simulink model "Shin_com"  (R2024a)
settings: Solver=VariableStepAuto  StartTime=0.0  StopTime=10.0  RelTol=1e-3
undefined symbols (not defined in the file): route1_waypoint_x, route1_waypoint_y, route2_waypoint_x, route2_waypoint_y, route3_waypoint_x, route3_waypoint_y, route4_waypoint_x, route4_waypoint_y, route5_waypoint_x, route5_waypoint_y
libraries: CarMaker4SL x162, slpidlib x4, robotalgslib x1, matrix_library x1
(part 1 of 4)
settings Model: Creator=User  LastModifiedBy=User

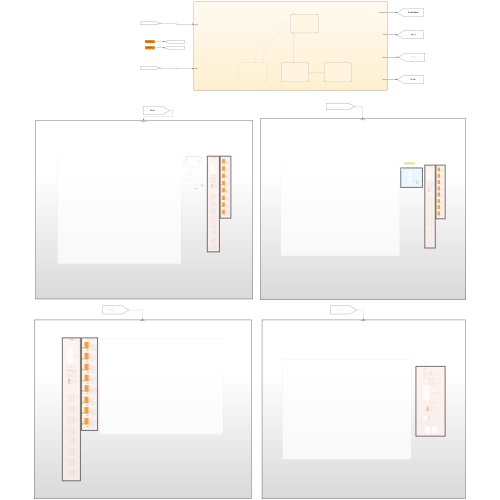
[thumbnail: Simulink's stored preview of the top-level diagram]
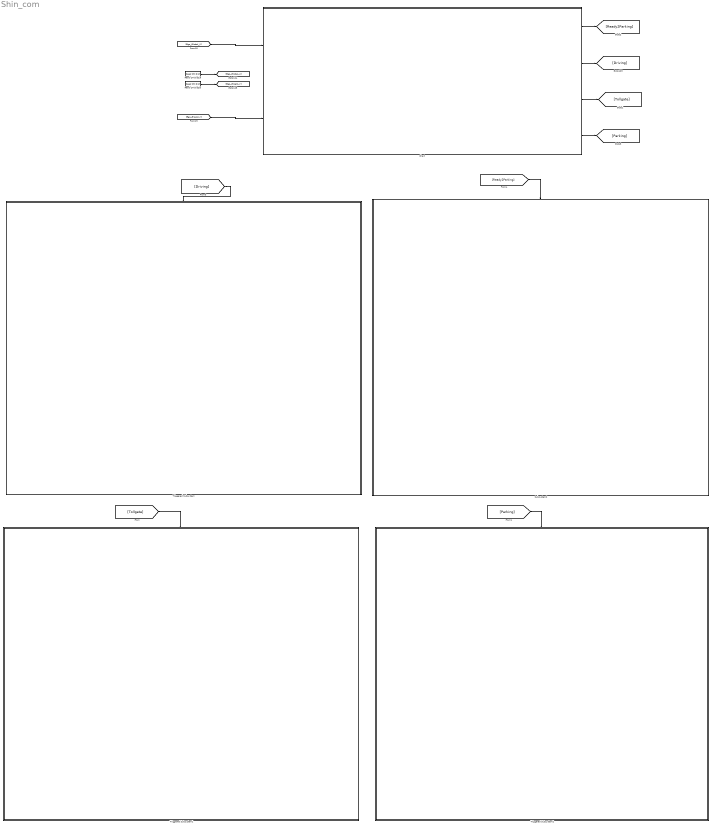
== system Shin_com ==
  Chart : Stateflow chart  TreatAsAtomicUnit=on
  Read CM Dict19 : CarMaker4SL/Read CM Dict  xname=Car.Fr1.tx  xsync=off  xstime=Inherited
  Read CM Dict20 : CarMaker4SL/Read CM Dict  xname=Car.Fr1.ty  xsync=off  xstime=Inherited
  Subsystem2 : Subsystem
  Triggered Subsystem : Subsystem  TreatAsAtomicUnit=on
  Triggered Subsystem1 : Subsystem  TreatAsAtomicUnit=on
  Triggered Subsystem2 : Subsystem  TreatAsAtomicUnit=on
  wires:
  Chart/3(tollgate()) -> [Tollgate]
  Read CM Dict20/1 -> [Ego_Gloabl_Y]
  [Driving] -> Triggered Subsystem/Trigger
  Chart/1(ready2parking()) -> [Ready2Parking]
  Chart/2(driving()) -> [Driving]
  [Ready2Parking] -> Subsystem2/Trigger
  [Ego_Global_X] -> Chart/1(global_X)
  [Ego_Gloabl_Y] -> Chart/2(global_Y)
  [Parking] -> Triggered Subsystem2/Trigger
  Chart/4(parking()) -> [Parking]
  Read CM Dict19/1 -> [Ego_Global_X]
  [Tollgate] -> Triggered Subsystem1/Trigger

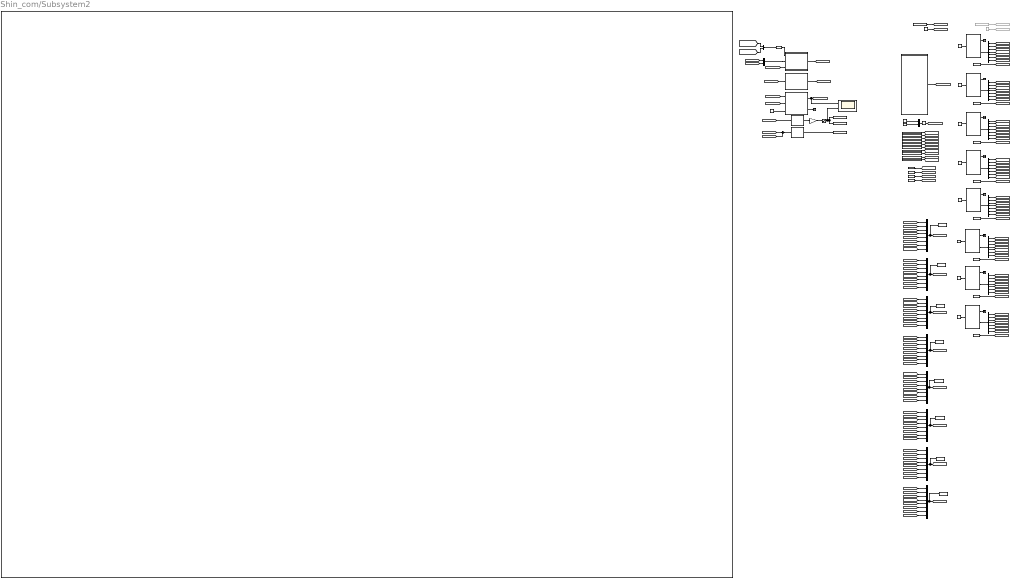
== system Shin_com/Subsystem2 ==
  note: Rpute 5
  note: *** Final Project ***
      |
      | Scenario:
      | Input:
      | Output:
      | 제어기 10ms / 다익스트라 1s
  note: Traffic Size
      | Length: 4.47
      | Width: 1.97
      | Height: 1.12
  note: Traffic Size
      | Length: 4.47
      | Width: 1.97
      | Height: 1.12
  note: Traffic Size
      | Length: 4.47
      | Width: 1.97
      | Height: 1.12
  note: Traffic Size
      | Length: 4.47
      | Width: 1.97
      | Height: 1.12
  note: Do Not Modify !!
  note: Traffic Size
      | Length: 4.47
      | Width: 1.97
      | Height: 1.12
  note: Traffic Size
      | Length: 4.47
      | Width: 1.97
      | Height: 1.12
  note: Do Not Modify !!
  note: Traffic Size
      | Length: 4.47
      | Width: 1.97
      | Height: 1.12
  note: Traffic Size
      | Length: 4.47
      | Width: 1.97
      | Height: 1.12
  Trigger : TriggerPort  TriggerType=function-call  VariantControl=(inherit)  PortDimensions=1
      mask Display: image('20210726111455075uqcv.jpg');
  Bus Selector{3..10} (8 alike) : BusSelector  OutputSignals=t_0 x,t_0 y,v_0 x,v_0 y,a_0 x,a_0 y,r_zyx z
  Constant : Constant  Value=0.5
  Constant11 : Constant  Value=28
  Constant12 : Constant  Value=route1_waypoint_y.Data
  Constant13 : Constant  Value=route2_waypoint_y.Data
  Constant14 : Constant  Value=route2_waypoint_x.Data
  Constant15 : Constant  Value=route1_waypoint_x.Data
  Constant16 : Constant  Value=route3_waypoint_y.Data
  Constant17 : Constant  Value=route3_waypoint_x.Data
  Constant18 : Constant  Value=route4_waypoint_y.Data
  Constant19 : Constant  Value=route4_waypoint_x.Data
  Constant20 : Constant  Value=route5_waypoint_y.Data
  Constant21 : Constant  Value=route5_waypoint_x.Data
  Constant22 : Constant  Value=23
  Constant23 : Constant  Value=20/3.6
  Constant25 : Constant  Value=11.5
  Constant26 : Constant  Value=24
  Constant27 : Constant  Value=25
  Constant28 : Constant  Value=26
  Constant29 : Constant  Value=27
  Constant6 : Constant  Commented=on  Value=20/3.6
  Constant7 : Constant  Value=21
  Constant8 : Constant  Value=2.48
  Constant9 : Constant  Value=22
  Gain : Gain  Gain=pi/180
  Goto31 : Goto  Commented=on  GotoTag=CrossTrackError
  Goto64 : Goto  Commented=on  GotoTag=Target_Speed
  MATLAB Function4 : MATLAB Function  TreatAsAtomicUnit=on
  "MATLAB Function4 " : MATLAB Function  TreatAsAtomicUnit=on
  MATLAB Function7 : MATLAB Function  TreatAsAtomicUnit=on
  Mux{,1..2,5..9} (8 alike) : Mux  Inputs=8
  Mux12 : Mux  Inputs=2
  Mux13 : Mux  Inputs=2
  Mux4 : Mux  Inputs=2
  PID Controller2 : slpidlib/PID Controller  Controller=PID  Form=Parallel  TimeDomain=Discrete-time  UseExternalTs=off  SampleTime=-1  IntegratorMethod=Forward Euler  FilterMethod=Forward Euler  ControllerParametersSource=internal  P=1  I=0.0  UseKiTs=off  D=0  UseExternalDerivativeSource=off  N=100  UseFilter=on  TunerSelectOption=Transfer Function Based (PID Tuner App)  InitialConditionSource=internal  InitialConditionForIntegrator=0  InitialConditionForFilter=0  DifferentiatorICPrevScaledInput=0  ExternalReset=none  TrackingMode=off  Kt=1  LimitOutput=off  SatLimitsSource=internal  UpperSaturationLimit=inf  LowerSaturationLimit=-inf  LinearizeAsGain=on  AntiWindupMode=none  Kb=1  LimitIntegrator=off  UpperIntegratorSaturationLimit=inf  LowerIntegratorSaturationLimit=-inf  POutMin=[]  POutMax=[]  IOutMin=[]  IOutMax=[]  DOutMin=[]  DOutMax=[]  NOutMin=[]  NOutMax=[]  SumOutMin=[]  SumOutMax=[]  SaturationOutMin=[]  SaturationOutMax=[]  PParamMin=[]  PParamMax=[]  IParamMin=[]  IParamMax=[]  DParamMin=[]  DParamMax=[]  NParamMin=[]  NParamMax=[]  KbParamMin=[]  KbParamMax=[]  KtParamMin=[]  KtParamMax=[]  KbOutMin=[]  KbOutMax=[]  KtOutMin=[]  KtOutMax=[]  IntegratorOutMin=[]  IntegratorOutMax=[]  FilterOutMin=[]  FilterOutMax=[]  SumI1OutMin=[]  SumI1OutMax=[]  SumI2OutMin=[]  SumI2OutMax=[]  SumI3OutMin=[]  SumI3OutMax=[]  SumI4OutMin=[]  SumI4OutMax=[]  SumDOutMin=[]  SumDOutMax=[]  DifferentiatorOutMin=[]  DifferentiatorOutMax=[]  FilterDiffOutCoefMin=[]  FilterDiffOutCoefMax=[]  ReciprocalOutMin=[]  ReciprocalOutMax=[]  SumDenOutMin=[]  SumDenOutMax=[]  SumNumOutMin=[]  SumNumOutMax=[]  DivideOutMin=[]  DivideOutMax=[]  UdiffTsProdOutMin=[]  UdiffTsProdOutMax=[]  NTsProdOutMin=[]  NTsProdOutMax=[]  UintegralTsProdOutMin=[]  UintegralTsProdOutMax=[]  UngainTsProdOutMin=[]  UngainTsProdOutMax=[]  ClampingZeroOutDataTypeStr=Inherit: Inherit via back propagation  ClampingZeroOutMin=[]  ClampingZeroOutMax=[]  FilterDenConstantOutDataTypeStr=Inherit: Inherit via back propagation  FilterDenConstantOutMin=[]  FilterDenConstantOutMax=[]  PCopyOutDataTypeStr=Inherit: Inherit via back propagation  PCopyOutMin=[]  PCopyOutMax=[]  NCopyOutDataTypeStr=Inherit: Inherit via back propagation  NCopyOutMin=[]  NCopyOutMax=[]  IntegratorContinuousStateAttributes=''  IntegratorStateMustResolveToSignalObject=off  IntegratorRTWStateStorageClass=Auto  FilterContinuousStateAttributes=''  FilterStateMustResolveToSignalObject=off  FilterRTWStateStorageClass=Auto  ParallelPVariant=InternalParameters  IdealPVariant=Disabled  IVariant=InternalParameters  DVariant=InternalParameters  IntegratorVariant=Discrete  SatVariant=Disabled  AWVariant=Passthrough  PCopyVariant=Disabled  TRVariant=Disabled  FdbkBlocksVariant=Forward  IdealPFdbkVariant=Disabled  SatFdbkVariant=Disabled  DerivativeFilterVariant=ForwardEulerFilter  NVariant=InternalParameters  NCopyVariant=Disabled  FilterICVariant=InternalICsFilter  IntegratorICVariant=InternalICs  ExternalResetVariant=Disabled  TRSumVariant=Passthrough  SumFdbkVariant=Disabled  SumVariant=Sum_PID  TsampFilterVariant=InternalTs  TsampNgainVariant=Passthrough  TsampIntegralVariant=Disabled_SignalSpec  ExternalSaturationOutDataTypeStr=Inherit: Same as second input  DerivativeSourceVariant=ErrorSignal
  PID Controller3 : slpidlib/PID Controller  Controller=PID  Form=Parallel  TimeDomain=Discrete-time  UseExternalTs=off  SampleTime=-1  IntegratorMethod=Forward Euler  FilterMethod=Forward Euler  ControllerParametersSource=internal  P=10  I=0  UseKiTs=off  D=0.1  UseExternalDerivativeSource=off  N=20  UseFilter=on  TunerSelectOption=Transfer Function Based (PID Tuner App)  InitialConditionSource=internal  InitialConditionForIntegrator=0  InitialConditionForFilter=0  DifferentiatorICPrevScaledInput=0  ExternalReset=none  TrackingMode=off  Kt=1  LimitOutput=off  SatLimitsSource=internal  UpperSaturationLimit=inf  LowerSaturationLimit=-inf  LinearizeAsGain=on  AntiWindupMode=none  Kb=1  LimitIntegrator=off  UpperIntegratorSaturationLimit=inf  LowerIntegratorSaturationLimit=-inf  POutMin=[]  POutMax=[]  IOutMin=[]  IOutMax=[]  DOutMin=[]  DOutMax=[]  NOutMin=[]  NOutMax=[]  SumOutMin=[]  SumOutMax=[]  SaturationOutMin=[]  SaturationOutMax=[]  PParamMin=[]  PParamMax=[]  IParamMin=[]  IParamMax=[]  DParamMin=[]  DParamMax=[]  NParamMin=[]  NParamMax=[]  KbParamMin=[]  KbParamMax=[]  KtParamMin=[]  KtParamMax=[]  KbOutMin=[]  KbOutMax=[]  KtOutMin=[]  KtOutMax=[]  IntegratorOutMin=[]  IntegratorOutMax=[]  FilterOutMin=[]  FilterOutMax=[]  SumI1OutMin=[]  SumI1OutMax=[]  SumI2OutMin=[]  SumI2OutMax=[]  SumI3OutMin=[]  SumI3OutMax=[]  SumI4OutMin=[]  SumI4OutMax=[]  SumDOutMin=[]  SumDOutMax=[]  DifferentiatorOutMin=[]  DifferentiatorOutMax=[]  FilterDiffOutCoefMin=[]  FilterDiffOutCoefMax=[]  ReciprocalOutMin=[]  ReciprocalOutMax=[]  SumDenOutMin=[]  SumDenOutMax=[]  SumNumOutMin=[]  SumNumOutMax=[]  DivideOutMin=[]  DivideOutMax=[]  UdiffTsProdOutMin=[]  UdiffTsProdOutMax=[]  NTsProdOutMin=[]  NTsProdOutMax=[]  UintegralTsProdOutMin=[]  UintegralTsProdOutMax=[]  UngainTsProdOutMin=[]  UngainTsProdOutMax=[]  ClampingZeroOutDataTypeStr=Inherit: Inherit via back propagation  ClampingZeroOutMin=[]  ClampingZeroOutMax=[]  FilterDenConstantOutDataTypeStr=Inherit: Inherit via back propagation  FilterDenConstantOutMin=[]  FilterDenConstantOutMax=[]  PCopyOutDataTypeStr=Inherit: Inherit via back propagation  PCopyOutMin=[]  PCopyOutMax=[]  NCopyOutDataTypeStr=Inherit: Inherit via back propagation  NCopyOutMin=[]  NCopyOutMax=[]  IntegratorContinuousStateAttributes=''  IntegratorStateMustResolveToSignalObject=off  IntegratorRTWStateStorageClass=Auto  FilterContinuousStateAttributes=''  FilterStateMustResolveToSignalObject=off  FilterRTWStateStorageClass=Auto  ParallelPVariant=InternalParameters  IdealPVariant=Disabled  IVariant=InternalParameters  DVariant=InternalParameters  IntegratorVariant=Discrete  SatVariant=Disabled  AWVariant=Passthrough  PCopyVariant=Disabled  TRVariant=Disabled  FdbkBlocksVariant=Forward  IdealPFdbkVariant=Disabled  SatFdbkVariant=Disabled  DerivativeFilterVariant=ForwardEulerFilter  NVariant=InternalParameters  NCopyVariant=Disabled  FilterICVariant=InternalICsFilter  IntegratorICVariant=InternalICs  ExternalResetVariant=Disabled  TRSumVariant=Passthrough  SumFdbkVariant=Disabled  SumVariant=Sum_PID  TsampFilterVariant=InternalTs  TsampNgainVariant=Passthrough  TsampIntegralVariant=Disabled_SignalSpec  ExternalSaturationOutDataTypeStr=Inherit: Same as second input  DerivativeSourceVariant=ErrorSignal
  Read CM Dict10 : CarMaker4SL/Read CM Dict  xname=Car.Fr1.tx  xsync=off  xstime=Inherited
  Read CM Dict11 : CarMaker4SL/Read CM Dict  xname=Car.Fr1.ty  xsync=off  xstime=Inherited
  Read CM Dict12 : CarMaker4SL/Read CM Dict  xname=Car.Fr1.rz  xsync=off  xstime=Inherited
  Read CM Dict13 : CarMaker4SL/Read CM Dict  xname=Car.v  xsync=off  xstime=Inherited
  Read CM Dict14 : CarMaker4SL/Read CM Dict  xname=Traffic.T24.rzv  xsync=off  xstime=Inherited
  Read CM Dict15 : CarMaker4SL/Read CM Dict  xname=Traffic.T25.rzv  xsync=off  xstime=Inherited
  Read CM Dict16 : CarMaker4SL/Read CM Dict  xname=Traffic.T26.rzv  xsync=off  xstime=Inherited
  Read CM Dict17 : CarMaker4SL/Read CM Dict  xname=Traffic.T27.rzv  xsync=off  xstime=Inherited
  Read CM Dict18 : CarMaker4SL/Read CM Dict  xname=Traffic.T28.rzv  xsync=off  xstime=Inherited
  Read CM Dict5 : CarMaker4SL/Read CM Dict  Commented=on  xname=Car.Road.Path.DevDist  xsync=off  xstime=Inherited
  Read CM Dict6 : CarMaker4SL/Read CM Dict  xname=Traffic.T21.rzv  xsync=off  xstime=Inherited
  Read CM Dict7 : CarMaker4SL/Read CM Dict  xname=Traffic.T22.rzv  xsync=off  xstime=Inherited
  Read CM Dict8 : CarMaker4SL/Read CM Dict  xname=Traffic.T23.rzv  xsync=off  xstime=Inherited
  Read CM Dict9 : CarMaker4SL/Read CM Dict  xname=Car.Road.Path.DevDist  xsync=off  xstime=Inherited
  Reshape2 : Reshape  OutputDimensionality=Row vector (2-D)  OutputDimensions=[2,2]
  Reshape3 : Reshape  OutputDimensionality=Customize  OutputDimensions=[201, 2]
  Saturation1 : Saturate  UpperLimit=2  LowerLimit=-2
  Scope : Scope  NumInputPorts=2
  Subsystem1 : Subsystem
  Sum : Sum  Inputs=|+-
  Terminator{,3..9,11} (9 alike) : Terminator
  To Workspace : ToWorkspace  VariableName=obs_x2  SaveFormat=Timeseries  SampleTime=-1
  To Workspace1 : ToWorkspace  VariableName=obs_Vx2  SaveFormat=Timeseries  SampleTime=-1
  To Workspace2 : ToWorkspace  VariableName=obs_YawRate2  SaveFormat=Timeseries  SampleTime=-1
  To Workspace3 : ToWorkspace  VariableName=obs_Ax2  SaveFormat=Timeseries  SampleTime=-1
  To Workspace4 : ToWorkspace  VariableName=obs_y2  SaveFormat=Timeseries  SampleTime=-1
  To Workspace5 : ToWorkspace  VariableName=obs_Vy2  SaveFormat=Timeseries  SampleTime=-1
  To Workspace6 : ToWorkspace  VariableName=obs_Yaw2  SaveFormat=Timeseries  SampleTime=-1
  To Workspace7 : ToWorkspace  VariableName=obs_Ay2  SaveFormat=Timeseries  SampleTime=-1
  Traffic Object10 : CarMaker4SL/Traffic Object  xname=T28  ximode=Traffic Id  xstime=Inherited
      settings: SourceProductName=CarMaker4SL
  Traffic Object3 : CarMaker4SL/Traffic Object  xname=T21  ximode=Traffic Id  xstime=Inherited
      settings: SourceProductName=CarMaker4SL
  Traffic Object4 : CarMaker4SL/Traffic Object  xname=T22  ximode=Traffic Id  xstime=Inherited
      settings: SourceProductName=CarMaker4SL
  Traffic Object5 : CarMaker4SL/Traffic Object  xname=T23  ximode=Traffic Id  xstime=Inherited
      settings: SourceProductName=CarMaker4SL
  Traffic Object6 : CarMaker4SL/Traffic Object  xname=T24  ximode=Traffic Id  xstime=Inherited
      settings: SourceProductName=CarMaker4SL
  Traffic Object7 : CarMaker4SL/Traffic Object  xname=T25  ximode=Traffic Id  xstime=Inherited
      settings: SourceProductName=CarMaker4SL
  Traffic Object8 : CarMaker4SL/Traffic Object  xname=T26  ximode=Traffic Id  xstime=Inherited
      settings: SourceProductName=CarMaker4SL
  Traffic Object9 : CarMaker4SL/Traffic Object  xname=T27  ximode=Traffic Id  xstime=Inherited
      settings: SourceProductName=CarMaker4SL
  Write CM Dict1 : CarMaker4SL/Write CM Dict  xname=AccelCtrl.DesiredAx  xsync=off
  Write CM Dict2 : CarMaker4SL/Write CM Dict  xname=Car.CFL.rz_ext  xsync=off
  Write CM Dict3 : CarMaker4SL/Write CM Dict  xname=Car.CFR.rz_ext  xsync=off
  wires:
  [Ego_Gloabl_Y] -> Mux13/2
  Mux12/1 -> Reshape3/1
  Reshape3/1 -> "MATLAB Function4 "/1(waypoints)
  [Ego_Global_X] -> Mux13/1
  [route5_waypoint_x] -> Mux12/1
  "MATLAB Function4 "/1(local_waypoints_) -> [Local_Points]
  [route5_waypoint_y] -> Mux12/2
  Mux13/1 -> "MATLAB Function4 "/2(vehicle_position)
  [Ego_Yaw] -> "MATLAB Function4 "/3(head)
  MATLAB Function7/1(poly_coeff) -> [Coefficients]
  [Local_Points] -> MATLAB Function7/1(local_waypoints)
  [Coefficients] -> MATLAB Function4/1(poly_coeff)
  MATLAB Function4/1(lateral_error) -> Scope/1, [LateralError]  "LatelralError"
  [LateralError] -> PID Controller3/1
  [Traffic27_Ax] -> Mux8/7
  Bus Selector10/1 -> [Traffic28_Global_X]  "<t_0 x>"
  Constant25/1 -> Mux4/2
  [Traffic23_Ay] -> Mux9/3
  [Traffic25_Yaw] -> Mux7/5
  Constant7/1 -> Traffic Object3/1
  Read CM Dict15/1 -> [Traffic25_YawRate]
  [Traffic23_Ax] -> Mux8/3
  Bus Selector6/3 -> [Traffic24_Vx]  "<v_0 x>"
  [Traffic23_Vy] -> Mux5/3
  Bus Selector7/5 -> [Traffic25_Ax]  "<a_0 x>"
  Bus Selector10/3 -> [Traffic28_Vx]  "<v_0 x>"
  Bus Selector3/6 -> [Traffic21_Ay]  "<a_0 y>"
  Constant20/1 -> [route5_waypoint_y]
  Constant27/1 -> Traffic Object7/1
  [Traffic26_Yaw] -> Mux7/6
  Subsystem1/1(Traffic_Info) -> [Traffic_Info]
  Bus Selector8/2 -> [Traffic26_Global_Y]  "<t_0 y>"
  Constant9/1 -> Traffic Object4/1
  Mux8/1 -> To Workspace3/1, [obs_Ax]
  Constant21/1 -> [route5_waypoint_x]
  Bus Selector5/4 -> [Traffic23_Vy]  "<v_0 y>"
  Read CM Dict7/1 -> [Traffic22_YawRate]
  Bus Selector7/3 -> [Traffic25_Vx]  "<v_0 x>"
  [Traffic25_Vx] -> Mux2/5
  Constant16/1 -> [route3_waypoint_y]
  Constant18/1 -> [route4_waypoint_y]
  [Traffic27_Vy] -> Mux5/7
  Traffic Object8/1 -> Terminator8/1
  [Traffic23_Global_X] -> Mux/3
  Constant19/1 -> [route4_waypoint_x]
  [Traffic21_Global_X] -> Mux/1
  Traffic Object4/2 -> Bus Selector4/1
  [Traffic25_YawRate] -> Mux6/5
  Bus Selector9/5 -> [Traffic27_Ax]  "<a_0 x>"
  Bus Selector8/5 -> [Traffic26_Ax]  "<a_0 x>"
  Read CM Dict11/1 -> [Ego_Gloabl_Y]
  [Traffic28_Global_X] -> Mux/8
  Read CM Dict16/1 -> [Traffic26_YawRate]
  Traffic Object6/1 -> Terminator6/1
  [Traffic28_Global_Y] -> Mux1/8
  Mux2/1 -> To Workspace1/1, [obs_Vx]
  [Traffic24_Vx] -> Mux2/4
  Constant17/1 -> [route3_waypoint_x]
  [Traffic25_Vy] -> Mux5/5
  [Traffic21_Vx] -> Mux2/1
  Read CM Dict6/1 -> [Traffic21_YawRate]
  [Traffic21_Ay] -> Mux9/1
  [Traffic23_Yaw] -> Mux7/3
  Constant8/1 -> Mux4/1
  [Traffic24_Yaw] -> Mux7/4
  Traffic Object10/2 -> Bus Selector10/1
  Mux5/1 -> To Workspace5/1, [obs_Vy]
  Bus Selector7/7 -> [Traffic25_Yaw]  "<r_zyx z>"
  Traffic Object8/2 -> Bus Selector8/1
  Bus Selector10/5 -> [Traffic28_Ax]  "<a_0 x>"
  [Traffic28_Vx] -> Mux6/8
  [Traffic27_YawRate] -> Mux6/7
  Read CM Dict10/1 -> [Ego_Global_X]
  [Traffic23_Global_Y] -> Mux1/3
  Bus Selector10/6 -> [Traffic28_Ay]  "<a_0 y>"
  [Traffic27_Ay] -> Mux9/7
  [Traffic26_Global_X] -> Mux/6
  Read CM Dict17/1 -> [Traffic27_YawRate]
  [Traffic24_Ax] -> Mux8/4
  Bus Selector6/6 -> [Traffic24_Ay]  "<a_0 y>"
  [Traffic24_Global_X] -> Mux/4
  [Traffic23_YawRate] -> Mux6/3
  Bus Selector10/4 -> [Traffic28_Vy]  "<v_0 y>"
  [Traffic27_Global_Y] -> Mux1/7
  Bus Selector3/4 -> [Traffic21_Vy]  "<v_0 y>"
  Bus Selector3/1 -> [Traffic21_Global_X]  "<t_0 x>"
  [Traffic24_Global_Y] -> Mux1/4
  [Traffic28_Vx] -> Mux2/8
  Bus Selector9/6 -> [Traffic27_Ay]  "<a_0 y>"
  Bus Selector8/3 -> [Traffic26_Vx]  "<v_0 x>"
  Bus Selector10/7 -> [Traffic28_Yaw]  "<r_zyx z>"
  Constant14/1 -> [route2_waypoint_x]
  Constant15/1 -> [route1_waypoint_x]
  Bus Selector7/6 -> [Traffic25_Ay]  "<a_0 y>"
  Constant6/1 -> Goto64/1
  Traffic Object6/2 -> Bus Selector6/1
  Mux7/1 -> To Workspace6/1, [obs_Yaw]
  [Traffic26_Ax] -> Mux8/6
  [Traffic27_Yaw] -> Mux7/7
  Bus Selector9/3 -> [Traffic27_Vx]  "<v_0 x>"
  Bus Selector4/4 -> [Traffic22_Vy]  "<v_0 y>"
  Bus Selector4/2 -> [Traffic22_Global_Y]  "<t_0 y>"
  [Traffic28_Yaw] -> Mux7/8
  [Traffic24_Vy] -> Mux5/4
  Bus Selector4/1 -> [Traffic22_Global_X]  "<t_0 x>"
  Bus Selector4/6 -> [Traffic22_Ay]  "<a_0 y>"
  Bus Selector4/3 -> [Traffic22_Vx]  "<v_0 x>"
  [Traffic22_Ay] -> Mux9/2
  [Traffic25_Ay] -> Mux9/5
  Traffic Object9/1 -> Terminator9/1
  [Traffic25_Ax] -> Mux8/5
  Constant28/1 -> Traffic Object8/1
  Mux9/1 -> To Workspace7/1, [obs_Ay]
  Traffic Object9/2 -> Bus Selector9/1
  [Traffic21_Vy] -> Mux5/1
  Bus Selector5/1 -> [Traffic23_Global_X]  "<t_0 x>"
  Bus Selector5/3 -> [Traffic23_Vx]  "<v_0 x>"
  Bus Selector9/7 -> [Traffic27_Yaw]  "<r_zyx z>"
  Constant22/1 -> Traffic Object5/1
  Bus Selector7/2 -> [Traffic25_Global_Y]  "<t_0 y>"
  [Traffic22_Vx] -> Mux2/2
  Traffic Object10/1 -> Terminator11/1
  Bus Selector6/4 -> [Traffic24_Vy]  "<v_0 y>"
  Traffic Object3/2 -> Bus Selector3/1
  Constant26/1 -> Traffic Object6/1
  Traffic Object7/2 -> Bus Selector7/1
  Read CM Dict9/1 -> [CrossTrackError]
  [Traffic21_YawRate] -> Mux6/1
  Bus Selector4/7 -> [Traffic22_Yaw]  "<r_zyx z>"
  Read CM Dict8/1 -> [Traffic23_YawRate]
  Bus Selector7/1 -> [Traffic25_Global_X]  "<t_0 x>"
  Bus Selector3/5 -> [Traffic21_Ax]  "<a_0 x>"
  Traffic Object4/1 -> Terminator4/1
  Traffic Object5/1 -> Terminator5/1
  [Traffic25_Global_Y] -> Mux1/5
  Read CM Dict18/1 -> [Traffic28_YawRate]
  [Traffic27_Vx] -> Mux2/7
  [Traffic28_Ay] -> Mux9/8
  Bus Selector5/5 -> [Traffic23_Ax]  "<a_0 x>"
  [Traffic27_Global_X] -> Mux/7
  Traffic Object3/1 -> Terminator3/1
  Mux/1 -> To Workspace/1, [obs_x]
  Mux1/1 -> To Workspace4/1, [obs_y]
  Bus Selector5/6 -> [Traffic23_Ay]  "<a_0 y>"
  [Traffic21_Yaw] -> Mux7/1
  [Traffic26_Ay] -> Mux9/6
  Traffic Object7/1 -> Terminator7/1
  Constant23/1 -> [Target_Speed]
  Bus Selector5/7 -> [Traffic23_Yaw]  "<r_zyx z>"
  [Traffic25_Global_X] -> Mux/5
  [Traffic22_Ax] -> Mux8/2
  Bus Selector8/4 -> [Traffic26_Vy]  "<v_0 y>"
  [Traffic26_Global_Y] -> Mux1/6
  Constant29/1 -> Traffic Object9/1
  Read CM Dict5/1 -> Goto31/1
  Bus Selector6/7 -> [Traffic24_Yaw]  "<r_zyx z>"
  [Traffic24_YawRate] -> Mux6/4
  Bus Selector5/2 -> [Traffic23_Global_Y]  "<t_0 y>"
  Bus Selector4/5 -> [Traffic22_Ax]  "<a_0 x>"
  Bus Selector6/2 -> [Traffic24_Global_Y]  "<t_0 y>"
  [Traffic26_Vx] -> Mux2/6
  [Traffic22_YawRate] -> Mux6/2
  Read CM Dict13/1 -> [Ego_Vx]
  [Traffic21_Ax] -> Mux8/1
  [Traffic22_Global_X] -> Mux/2
  [Traffic28_Ax] -> Mux8/8
  Bus Selector8/1 -> [Traffic26_Global_X]  "<t_0 x>"
  [Traffic22_Yaw] -> Mux7/2
  Constant11/1 -> Traffic Object10/1
  Bus Selector8/6 -> [Traffic26_Ay]  "<a_0 y>"
  Constant13/1 -> [route2_waypoint_y]
  Bus Selector9/1 -> [Traffic27_Global_X]  "<t_0 x>"
  Mux6/1 -> To Workspace2/1, [obs_YawRate]
  Bus Selector3/7 -> [Traffic21_Yaw]  "<r_zyx z>"
  Bus Selector9/2 -> [Traffic27_Global_Y]  "<t_0 y>"
  Bus Selector6/5 -> [Traffic24_Ax]  "<a_0 x>"
  Mux4/1 -> Reshape2/1
  [Traffic28_Vy] -> Mux5/8
  Bus Selector7/4 -> [Traffic25_Vy]  "<v_0 y>"
  Constant12/1 -> [route1_waypoint_y]
  Bus Selector9/4 -> [Traffic27_Vy]  "<v_0 y>"
  Reshape2/1 -> [Traffic_size]
  Read CM Dict12/1 -> [Ego_Yaw]
  Bus Selector3/3 -> [Traffic21_Vx]  "<v_0 x>"
  Bus Selector8/7 -> [Traffic26_Yaw]  "<r_zyx z>"
  [Traffic23_Vx] -> Mux2/3
  [Traffic22_Vy] -> Mux5/2
  [Traffic26_YawRate] -> Mux6/6
  [Traffic26_Vy] -> Mux5/6
  Traffic Object5/2 -> Bus Selector5/1
  [Traffic22_Global_Y] -> Mux1/2
  [Traffic21_Global_Y] -> Mux1/1
  Bus Selector3/2 -> [Traffic21_Global_Y]  "<t_0 y>"
  Bus Selector6/1 -> [Traffic24_Global_X]  "<t_0 x>"
  Read CM Dict14/1 -> [Traffic24_YawRate]
  [Traffic24_Ay] -> Mux9/4
  Bus Selector10/2 -> [Traffic28_Global_Y]  "<t_0 y>"
  [Ego_Vx] -> MATLAB Function4/2(velocity)
  Constant/1 -> MATLAB Function4/3(lookahead_time)
  MATLAB Function4/2(x_lookahead) -> Terminator/1
  PID Controller3/1 -> Gain/1
  Gain/1 -> Saturation1/1
  Saturation1/1 -> Scope/2, Write CM Dict3/1, Write CM Dict2/1  "Wheel Angle"
  [Target_Speed] -> Sum/1
  [Ego_Vx] -> Sum/2
  Sum/1 -> PID Controller2/1
  PID Controller2/1 -> Write CM Dict1/1  "Accel"

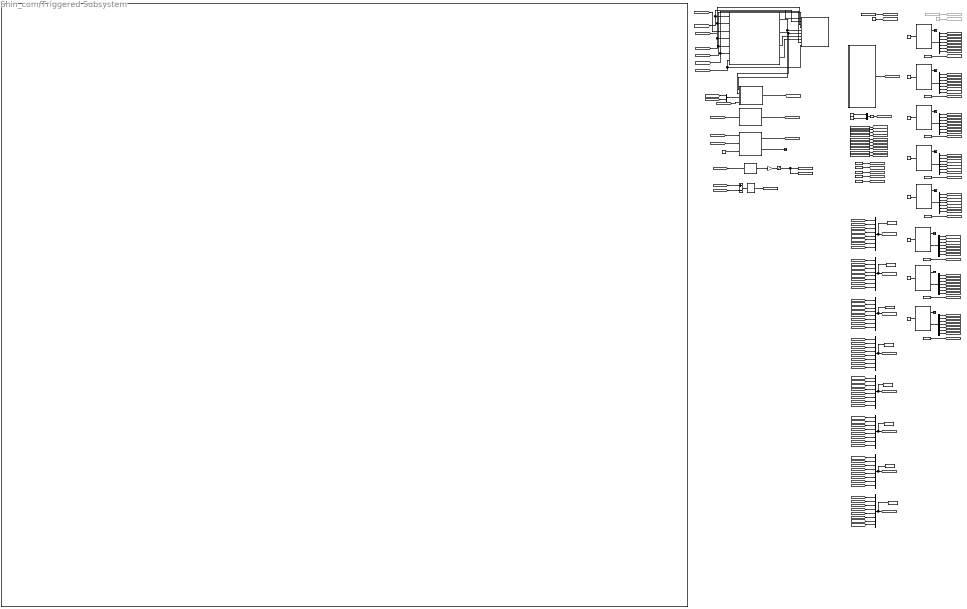
== system Shin_com/Triggered Subsystem ==
  note: Traffic Size
      | Length: 4.47
      | Width: 1.97
      | Height: 1.12
  note: Traffic Size
      | Length: 4.47
      | Width: 1.97
      | Height: 1.12
  note: Do Not Modify !!
  note: Traffic Size
      | Length: 4.47
      | Width: 1.97
      | Height: 1.12
  note: Do Not Modify !!
  note: Traffic Size
      | Length: 4.47
      | Width: 1.97
      | Height: 1.12
  note: Traffic Size
      | Length: 4.47
      | Width: 1.97
      | Height: 1.12
  note: Traffic Size
      | Length: 4.47
      | Width: 1.97
      | Height: 1.12
  note: Traffic Size
      | Length: 4.47
      | Width: 1.97
      | Height: 1.12
  note: Traffic Size
      | Length: 4.47
      | Width: 1.97
      | Height: 1.12
  Trigger : TriggerPort  TriggerType=function-call  VariantControl=(inherit)
      mask Display: image('KakaoTalk_20250521_160448332.jpg');
  Add : Sum  Inputs=+-
  Bus Selector{3..10} (8 alike) : BusSelector  OutputSignals=t_0 x,t_0 y,v_0 x,v_0 y,a_0 x,a_0 y,r_zyx z
  Constant11 : Constant  Value=28
  Constant12 : Constant  Value=route1_waypoint_y.Data
  Constant13 : Constant  Value=route2_waypoint_y.Data
  Constant14 : Constant  Value=route2_waypoint_x.Data
  Constant15 : Constant  Value=route1_waypoint_x.Data
  Constant16 : Constant  Value=route3_waypoint_y.Data
  Constant17 : Constant  Value=route3_waypoint_x.Data
  Constant18 : Constant  Value=route4_waypoint_y.Data
  Constant19 : Constant  Value=route4_waypoint_x.Data
  Constant20 : Constant  Value=route5_waypoint_y.Data
  Constant21 : Constant  Value=route5_waypoint_x.Data
  Constant22 : Constant  Value=23
  Constant23 : Constant  Value=30/3.6
  Constant25 : Constant  Value=11.5
  Constant26 : Constant  Value=24
  Constant27 : Constant  Value=25
  Constant28 : Constant  Value=26
  Constant29 : Constant  Value=27
  Constant30 : Constant  Value=0.5
  Constant6 : Constant  Commented=on  Value=20/3.6
  Constant7 : Constant  Value=21
  Constant8 : Constant  Value=2.48
  Constant9 : Constant  Value=22
  Gain2 : Gain  Gain=pi/180
  Goto31 : Goto  Commented=on  GotoTag=CrossTrackError
  Goto64 : Goto  Commented=on  GotoTag=Target_Speed
  MATLAB Function3 : MATLAB Function  TreatAsAtomicUnit=on
  MATLAB Function4 1 : MATLAB Function  TreatAsAtomicUnit=on
  MATLAB Function5 : MATLAB Function  TreatAsAtomicUnit=on
  MATLAB Function8 : MATLAB Function  TreatAsAtomicUnit=on
  MATLAB System : MATLABSystem  System=BasicTrajectoryViewerWithLanes  SimulateUsing=Interpreted execution
      mask Type: BasicTrajectoryViewerWithLanes
      mask Display:
      | disp('BasicTrajectoryViewerWithLanes');
      | port_label('input',1,'x');
      | port_label('input',2,'y');
      | port_label('input',3,'map_x');
      | port_label('input',4,'map_y');
      | port_label('input',5,'x_best');
      | port_label('input',6,'y_best');
      | port_label('input',7,'x_all');
      | port_label('input',8,'y_all');
      | port_label('input',9,'obs_x');
      | port_label('input',10,'obs_y');
  Mux{,1..2,5..9} (8 alike) : Mux  Inputs=8
  Mux11 : Mux  Inputs=2
  Mux4 : Mux  Inputs=2
  PID Controller : slpidlib/PID Controller  Controller=PID  Form=Parallel  TimeDomain=Discrete-time  UseExternalTs=off  SampleTime=-1  IntegratorMethod=Forward Euler  FilterMethod=Forward Euler  ControllerParametersSource=internal  P=5  I=0.0  UseKiTs=off  D=0.0  UseExternalDerivativeSource=off  N=100  UseFilter=on  TunerSelectOption=Transfer Function Based (PID Tuner App)  InitialConditionSource=internal  InitialConditionForIntegrator=0  InitialConditionForFilter=0  DifferentiatorICPrevScaledInput=0  ExternalReset=none  TrackingMode=off  Kt=1  LimitOutput=off  SatLimitsSource=internal  UpperSaturationLimit=inf  LowerSaturationLimit=-inf  LinearizeAsGain=on  AntiWindupMode=none  Kb=1  LimitIntegrator=off  UpperIntegratorSaturationLimit=inf  LowerIntegratorSaturationLimit=-inf  POutMin=[]  POutMax=[]  IOutMin=[]  IOutMax=[]  DOutMin=[]  DOutMax=[]  NOutMin=[]  NOutMax=[]  SumOutMin=[]  SumOutMax=[]  SaturationOutMin=[]  SaturationOutMax=[]  PParamMin=[]  PParamMax=[]  IParamMin=[]  IParamMax=[]  DParamMin=[]  DParamMax=[]  NParamMin=[]  NParamMax=[]  KbParamMin=[]  KbParamMax=[]  KtParamMin=[]  KtParamMax=[]  KbOutMin=[]  KbOutMax=[]  KtOutMin=[]  KtOutMax=[]  IntegratorOutMin=[]  IntegratorOutMax=[]  FilterOutMin=[]  FilterOutMax=[]  SumI1OutMin=[]  SumI1OutMax=[]  SumI2OutMin=[]  SumI2OutMax=[]  SumI3OutMin=[]  SumI3OutMax=[]  SumI4OutMin=[]  SumI4OutMax=[]  SumDOutMin=[]  SumDOutMax=[]  DifferentiatorOutMin=[]  DifferentiatorOutMax=[]  FilterDiffOutCoefMin=[]  FilterDiffOutCoefMax=[]  ReciprocalOutMin=[]  ReciprocalOutMax=[]  SumDenOutMin=[]  SumDenOutMax=[]  SumNumOutMin=[]  SumNumOutMax=[]  DivideOutMin=[]  DivideOutMax=[]  UdiffTsProdOutMin=[]  UdiffTsProdOutMax=[]  NTsProdOutMin=[]  NTsProdOutMax=[]  UintegralTsProdOutMin=[]  UintegralTsProdOutMax=[]  UngainTsProdOutMin=[]  UngainTsProdOutMax=[]  ClampingZeroOutDataTypeStr=Inherit: Inherit via back propagation  ClampingZeroOutMin=[]  ClampingZeroOutMax=[]  FilterDenConstantOutDataTypeStr=Inherit: Inherit via back propagation  FilterDenConstantOutMin=[]  FilterDenConstantOutMax=[]  PCopyOutDataTypeStr=Inherit: Inherit via back propagation  PCopyOutMin=[]  PCopyOutMax=[]  NCopyOutDataTypeStr=Inherit: Inherit via back propagation  NCopyOutMin=[]  NCopyOutMax=[]  IntegratorContinuousStateAttributes=''  IntegratorStateMustResolveToSignalObject=off  IntegratorRTWStateStorageClass=Auto  FilterContinuousStateAttributes=''  FilterStateMustResolveToSignalObject=off  FilterRTWStateStorageClass=Auto  ParallelPVariant=InternalParameters  IdealPVariant=Disabled  IVariant=InternalParameters  DVariant=InternalParameters  IntegratorVariant=Discrete  SatVariant=Disabled  AWVariant=Passthrough  PCopyVariant=Disabled  TRVariant=Disabled  FdbkBlocksVariant=Forward  IdealPFdbkVariant=Disabled  SatFdbkVariant=Disabled  DerivativeFilterVariant=ForwardEulerFilter  NVariant=InternalParameters  NCopyVariant=Disabled  FilterICVariant=InternalICsFilter  IntegratorICVariant=InternalICs  ExternalResetVariant=Disabled  TRSumVariant=Passthrough  SumFdbkVariant=Disabled  SumVariant=Sum_PID  TsampFilterVariant=InternalTs  TsampNgainVariant=Passthrough  TsampIntegralVariant=Disabled_SignalSpec  ExternalSaturationOutDataTypeStr=Inherit: Same as second input  DerivativeSourceVariant=ErrorSignal
  PID Controller1 : slpidlib/PID Controller  Controller=PID  Form=Parallel  TimeDomain=Discrete-time  UseExternalTs=off  SampleTime=-1  IntegratorMethod=Forward Euler  FilterMethod=Forward Euler  ControllerParametersSource=internal  P=5  I=0  UseKiTs=off  D=0.1  UseExternalDerivativeSource=off  N=20  UseFilter=on  TunerSelectOption=Transfer Function Based (PID Tuner App)  InitialConditionSource=internal  InitialConditionForIntegrator=0  InitialConditionForFilter=0  DifferentiatorICPrevScaledInput=0  ExternalReset=none  TrackingMode=off  Kt=1  LimitOutput=off  SatLimitsSource=internal  UpperSaturationLimit=inf  LowerSaturationLimit=-inf  LinearizeAsGain=on  AntiWindupMode=none  Kb=1  LimitIntegrator=off  UpperIntegratorSaturationLimit=inf  LowerIntegratorSaturationLimit=-inf  POutMin=[]  POutMax=[]  IOutMin=[]  IOutMax=[]  DOutMin=[]  DOutMax=[]  NOutMin=[]  NOutMax=[]  SumOutMin=[]  SumOutMax=[]  SaturationOutMin=[]  SaturationOutMax=[]  PParamMin=[]  PParamMax=[]  IParamMin=[]  IParamMax=[]  DParamMin=[]  DParamMax=[]  NParamMin=[]  NParamMax=[]  KbParamMin=[]  KbParamMax=[]  KtParamMin=[]  KtParamMax=[]  KbOutMin=[]  KbOutMax=[]  KtOutMin=[]  KtOutMax=[]  IntegratorOutMin=[]  IntegratorOutMax=[]  FilterOutMin=[]  FilterOutMax=[]  SumI1OutMin=[]  SumI1OutMax=[]  SumI2OutMin=[]  SumI2OutMax=[]  SumI3OutMin=[]  SumI3OutMax=[]  SumI4OutMin=[]  SumI4OutMax=[]  SumDOutMin=[]  SumDOutMax=[]  DifferentiatorOutMin=[]  DifferentiatorOutMax=[]  FilterDiffOutCoefMin=[]  FilterDiffOutCoefMax=[]  ReciprocalOutMin=[]  ReciprocalOutMax=[]  SumDenOutMin=[]  SumDenOutMax=[]  SumNumOutMin=[]  SumNumOutMax=[]  DivideOutMin=[]  DivideOutMax=[]  UdiffTsProdOutMin=[]  UdiffTsProdOutMax=[]  NTsProdOutMin=[]  NTsProdOutMax=[]  UintegralTsProdOutMin=[]  UintegralTsProdOutMax=[]  UngainTsProdOutMin=[]  UngainTsProdOutMax=[]  ClampingZeroOutDataTypeStr=Inherit: Inherit via back propagation  ClampingZeroOutMin=[]  ClampingZeroOutMax=[]  FilterDenConstantOutDataTypeStr=Inherit: Inherit via back propagation  FilterDenConstantOutMin=[]  FilterDenConstantOutMax=[]  PCopyOutDataTypeStr=Inherit: Inherit via back propagation  PCopyOutMin=[]  PCopyOutMax=[]  NCopyOutDataTypeStr=Inherit: Inherit via back propagation  NCopyOutMin=[]  NCopyOutMax=[]  IntegratorContinuousStateAttributes=''  IntegratorStateMustResolveToSignalObject=off  IntegratorRTWStateStorageClass=Auto  FilterContinuousStateAttributes=''  FilterStateMustResolveToSignalObject=off  FilterRTWStateStorageClass=Auto  ParallelPVariant=InternalParameters  IdealPVariant=Disabled  IVariant=InternalParameters  DVariant=InternalParameters  IntegratorVariant=Discrete  SatVariant=Disabled  AWVariant=Passthrough  PCopyVariant=Disabled  TRVariant=Disabled  FdbkBlocksVariant=Forward  IdealPFdbkVariant=Disabled  SatFdbkVariant=Disabled  DerivativeFilterVariant=ForwardEulerFilter  NVariant=InternalParameters  NCopyVariant=Disabled  FilterICVariant=InternalICsFilter  IntegratorICVariant=InternalICs  ExternalResetVariant=Disabled  TRSumVariant=Passthrough  SumFdbkVariant=Disabled  SumVariant=Sum_PID  TsampFilterVariant=InternalTs  TsampNgainVariant=Passthrough  TsampIntegralVariant=Disabled_SignalSpec  ExternalSaturationOutDataTypeStr=Inherit: Same as second input  DerivativeSourceVariant=ErrorSignal
  Read CM Dict1 : CarMaker4SL/Read CM Dict  xname=Car.ax  xsync=off  xstime=Inherited
  Read CM Dict10 : CarMaker4SL/Read CM Dict  xname=Car.Fr1.tx  xsync=off  xstime=Inherited
  Read CM Dict11 : CarMaker4SL/Read CM Dict  xname=Car.Fr1.ty  xsync=off  xstime=Inherited
  Read CM Dict12 : CarMaker4SL/Read CM Dict  xname=Car.Fr1.rz  xsync=off  xstime=Inherited
  Read CM Dict13 : CarMaker4SL/Read CM Dict  xname=Car.v  xsync=off  xstime=Inherited
  Read CM Dict14 : CarMaker4SL/Read CM Dict  xname=Traffic.T24.rzv  xsync=off  xstime=Inherited
  Read CM Dict15 : CarMaker4SL/Read CM Dict  xname=Traffic.T25.rzv  xsync=off  xstime=Inherited
  Read CM Dict16 : CarMaker4SL/Read CM Dict  xname=Traffic.T26.rzv  xsync=off  xstime=Inherited
  Read CM Dict17 : CarMaker4SL/Read CM Dict  xname=Traffic.T27.rzv  xsync=off  xstime=Inherited
  Read CM Dict18 : CarMaker4SL/Read CM Dict  xname=Traffic.T28.rzv  xsync=off  xstime=Inherited
  Read CM Dict5 : CarMaker4SL/Read CM Dict  Commented=on  xname=Car.Road.Path.DevDist  xsync=off  xstime=Inherited
  Read CM Dict6 : CarMaker4SL/Read CM Dict  xname=Traffic.T21.rzv  xsync=off  xstime=Inherited
  Read CM Dict7 : CarMaker4SL/Read CM Dict  xname=Traffic.T22.rzv  xsync=off  xstime=Inherited
  Read CM Dict8 : CarMaker4SL/Read CM Dict  xname=Traffic.T23.rzv  xsync=off  xstime=Inherited
  Read CM Dict9 : CarMaker4SL/Read CM Dict  xname=Car.Road.Path.DevDist  xsync=off  xstime=Inherited
  Reshape2 : Reshape  OutputDimensionality=Row vector (2-D)  OutputDimensions=[2,2]
  Saturation3 : Saturate  UpperLimit=2  LowerLimit=-2
  Subsystem1 : Subsystem
  Terminator{3..9,11..12} (9 alike) : Terminator
  To Workspace : ToWorkspace  VariableName=obs_x1  SaveFormat=Timeseries  SampleTime=-1
  To Workspace1 : ToWorkspace  VariableName=obs_Vx1  SaveFormat=Timeseries  SampleTime=-1
  To Workspace2 : ToWorkspace  VariableName=obs_YawRate1  SaveFormat=Timeseries  SampleTime=-1
  To Workspace3 : ToWorkspace  VariableName=obs_Ax1  SaveFormat=Timeseries  SampleTime=-1
  To Workspace4 : ToWorkspace  VariableName=obs_y1  SaveFormat=Timeseries  SampleTime=-1
  To Workspace5 : ToWorkspace  VariableName=obs_Vy1  SaveFormat=Timeseries  SampleTime=-1
  To Workspace6 : ToWorkspace  VariableName=obs_Yaw1  SaveFormat=Timeseries  SampleTime=-1
  To Workspace7 : ToWorkspace  VariableName=obs_Ay1  SaveFormat=Timeseries  SampleTime=-1
  Traffic Object10 : CarMaker4SL/Traffic Object  xname=T28  ximode=Traffic Id  xstime=Inherited
      settings: SourceProductName=CarMaker4SL
  Traffic Object3 : CarMaker4SL/Traffic Object  xname=T21  ximode=Traffic Id  xstime=Inherited
      settings: SourceProductName=CarMaker4SL
  Traffic Object4 : CarMaker4SL/Traffic Object  xname=T22  ximode=Traffic Id  xstime=Inherited
      settings: SourceProductName=CarMaker4SL
  Traffic Object5 : CarMaker4SL/Traffic Object  xname=T23  ximode=Traffic Id  xstime=Inherited
      settings: SourceProductName=CarMaker4SL
  Traffic Object6 : CarMaker4SL/Traffic Object  xname=T24  ximode=Traffic Id  xstime=Inherited
      settings: SourceProductName=CarMaker4SL
  Traffic Object7 : CarMaker4SL/Traffic Object  xname=T25  ximode=Traffic Id  xstime=Inherited
      settings: SourceProductName=CarMaker4SL
  Traffic Object8 : CarMaker4SL/Traffic Object  xname=T26  ximode=Traffic Id  xstime=Inherited
      settings: SourceProductName=CarMaker4SL
  Traffic Object9 : CarMaker4SL/Traffic Object  xname=T27  ximode=Traffic Id  xstime=Inherited
      settings: SourceProductName=CarMaker4SL
  Write CM Dict10 : CarMaker4SL/Write CM Dict  xname=Car.CFR.rz_ext  xsync=off
  Write CM Dict3 : CarMaker4SL/Write CM Dict  xname=AccelCtrl.DesiredAx  xsync=off
  Write CM Dict9 : CarMaker4SL/Write CM Dict  xname=Car.CFL.rz_ext  xsync=off
  wires:
  Constant30/1 -> MATLAB Function3/3(lookahead_time)
  [LateralErrorA] -> PID Controller1/1
  [CoefficientsA] -> MATLAB Function3/1(poly_coeff)
  Saturation3/1 -> Write CM Dict10/1, Write CM Dict9/1
  MATLAB Function5/1(x_best) -> MATLAB Function4 1/1(waypoint_x), MATLAB System/5
  MATLAB Function3/1(lateral_error) -> [LateralErrorA]
  [Ego_Yaw] -> MATLAB Function4 1/4(head)
  [Ego_Vx] -> MATLAB Function3/2(velocity)
  [Ego_Gloabl_Y] -> MATLAB Function5/2(y), MATLAB System/2
  MATLAB Function5/3(x_all) -> MATLAB System/7
  MATLAB Function8/1(poly_coeff) -> [CoefficientsA]
  [Ego_Global_X] -> Mux11/1
  [obs_y] -> MATLAB Function5/7(obs_y), MATLAB System/10
  Add/1 -> PID Controller/1
  [route2_waypoint_y] -> MATLAB Function5/5(map_y), MATLAB System/4
  MATLAB Function5/2(y_best) -> MATLAB Function4 1/2(waypoint_y), MATLAB System/6
  [Local_PointsA] -> MATLAB Function8/1(local_waypoints)
  MATLAB Function3/2(x_lookahead) -> Terminator12/1
  [Ego_Global_X] -> MATLAB Function5/1(x), MATLAB System/1
  Mux11/1 -> MATLAB Function4 1/3(vehicle_position)
  PID Controller1/1 -> Gain2/1
  Gain2/1 -> Saturation3/1
  [Ego_Gloabl_Y] -> Mux11/2
  MATLAB Function4 1/1(local_waypoints_) -> [Local_PointsA]
  [route2_waypoint_x] -> MATLAB Function5/4(map_x), MATLAB System/3
  [obs_x] -> MATLAB Function5/6(obs_x), MATLAB System/9
  [Ego_Vx] -> MATLAB Function5/3(v)
  PID Controller/1 -> Write CM Dict3/1
  MATLAB Function5/4(y_all) -> MATLAB System/8
  Read CM Dict8/1 -> [Traffic23_YawRate]
  [Traffic23_Ay] -> Mux9/3
  [Traffic27_Yaw] -> Mux7/7
  [Traffic27_Ax] -> Mux8/7
  Bus Selector10/1 -> [Traffic28_Global_X]  "<t_0 x>"
  Constant25/1 -> Mux4/2
  [Traffic26_Vx] -> Mux2/6
  [Traffic26_Global_Y] -> Mux1/6
  Read CM Dict13/1 -> [Ego_Vx]
  Bus Selector4/5 -> [Traffic22_Ax]  "<a_0 x>"
  Bus Selector6/7 -> [Traffic24_Yaw]  "<r_zyx z>"
  [Traffic24_YawRate] -> Mux6/4
  [Traffic22_YawRate] -> Mux6/2
  Read CM Dict5/1 -> Goto31/1
  [Traffic21_Ax] -> Mux8/1
  Bus Selector6/2 -> [Traffic24_Global_Y]  "<t_0 y>"
  Bus Selector5/7 -> [Traffic23_Yaw]  "<r_zyx z>"
  Constant23/1 -> [Target_Speed]
  Traffic Object3/1 -> Terminator3/1
  Read CM Dict12/1 -> [Ego_Yaw]
  [Traffic21_Yaw] -> Mux7/1
  [Traffic22_Ax] -> Mux8/2
  [Traffic26_Ay] -> Mux9/6
  [Traffic21_Global_Y] -> Mux1/1
  Bus Selector5/6 -> [Traffic23_Ay]  "<a_0 y>"
  Bus Selector9/1 -> [Traffic27_Global_X]  "<t_0 x>"
  Read CM Dict18/1 -> [Traffic28_YawRate]
  [Traffic22_Global_X] -> Mux/2
  [Traffic25_Global_Y] -> Mux1/5
  [Traffic27_Vx] -> Mux2/7
  [Traffic27_Global_X] -> Mux/7
  Bus Selector5/5 -> [Traffic23_Ax]  "<a_0 x>"
  Bus Selector5/2 -> [Traffic23_Global_Y]  "<t_0 y>"
  [Traffic25_Global_X] -> Mux/5
  Bus Selector9/2 -> [Traffic27_Global_Y]  "<t_0 y>"
  Traffic Object4/1 -> Terminator4/1
  Constant11/1 -> Traffic Object10/1
  Constant29/1 -> Traffic Object9/1
  Traffic Object5/1 -> Terminator5/1
  Bus Selector3/5 -> [Traffic21_Ax]  "<a_0 x>"
  Bus Selector10/2 -> [Traffic28_Global_Y]  "<t_0 y>"
  Mux6/1 -> To Workspace2/1, [obs_YawRate]
  Bus Selector7/2 -> [Traffic25_Global_Y]  "<t_0 y>"
  Bus Selector7/1 -> [Traffic25_Global_X]  "<t_0 x>"
  Traffic Object10/1 -> Terminator11/1
  [Traffic22_Vx] -> Mux2/2
  Read CM Dict9/1 -> [CrossTrackError]
  Bus Selector6/5 -> [Traffic24_Ax]  "<a_0 x>"
  Mux/1 -> To Workspace/1, [obs_x]
  Bus Selector9/7 -> [Traffic27_Yaw]  "<r_zyx z>"
  Traffic Object3/2 -> Bus Selector3/1
  Traffic Object7/2 -> Bus Selector7/1
  [Traffic28_Vy] -> Mux5/8
  [Traffic25_Ax] -> Mux8/5
  Mux9/1 -> To Workspace7/1, [obs_Ay]
  Traffic Object9/1 -> Terminator9/1
  [Traffic25_Ay] -> Mux9/5
  Bus Selector4/3 -> [Traffic22_Vx]  "<v_0 x>"
  Constant28/1 -> Traffic Object8/1
  Bus Selector5/3 -> [Traffic23_Vx]  "<v_0 x>"
  [Traffic21_Vy] -> Mux5/1
  [Traffic24_Vy] -> Mux5/4
  [Traffic28_Ay] -> Mux9/8
  Bus Selector4/4 -> [Traffic22_Vy]  "<v_0 y>"
  Bus Selector4/2 -> [Traffic22_Global_Y]  "<t_0 y>"
  [Traffic21_YawRate] -> Mux6/1
  Bus Selector9/3 -> [Traffic27_Vx]  "<v_0 x>"
  Bus Selector4/6 -> [Traffic22_Ay]  "<a_0 y>"
  [Traffic28_Yaw] -> Mux7/8
  Bus Selector5/1 -> [Traffic23_Global_X]  "<t_0 x>"
  Mux7/1 -> To Workspace6/1, [obs_Yaw]
  [Traffic26_Ax] -> Mux8/6
  Bus Selector9/6 -> [Traffic27_Ay]  "<a_0 y>"
  Constant14/1 -> [route2_waypoint_x]
  Traffic Object6/2 -> Bus Selector6/1
  Bus Selector7/6 -> [Traffic25_Ay]  "<a_0 y>"
  Constant6/1 -> Goto64/1
  Bus Selector8/3 -> [Traffic26_Vx]  "<v_0 x>"
  Constant15/1 -> [route1_waypoint_x]
  Traffic Object9/2 -> Bus Selector9/1
  [Traffic28_Vx] -> Mux2/8
  Bus Selector8/4 -> [Traffic26_Vy]  "<v_0 y>"
  [Traffic27_Global_Y] -> Mux1/7
  Bus Selector10/4 -> [Traffic28_Vy]  "<v_0 y>"
  [Traffic24_Global_X] -> Mux/4
  [Traffic24_Ax] -> Mux8/4
  Read CM Dict17/1 -> [Traffic27_YawRate]
  Constant26/1 -> Traffic Object6/1
  [Traffic24_Global_Y] -> Mux1/4
  Bus Selector3/1 -> [Traffic21_Global_X]  "<t_0 x>"
  Bus Selector3/4 -> [Traffic21_Vy]  "<v_0 y>"
  Bus Selector8/7 -> [Traffic26_Yaw]  "<r_zyx z>"
  [Traffic26_Global_X] -> Mux/6
  Bus Selector6/4 -> [Traffic24_Vy]  "<v_0 y>"
  [Traffic27_Ay] -> Mux9/7
  [Traffic23_Global_Y] -> Mux1/3
  Bus Selector10/6 -> [Traffic28_Ay]  "<a_0 y>"
  Read CM Dict10/1 -> [Ego_Global_X]
  Bus Selector6/6 -> [Traffic24_Ay]  "<a_0 y>"
  Traffic Object7/1 -> Terminator7/1
  [Traffic28_Vx] -> Mux6/8
  Traffic Object8/2 -> Bus Selector8/1
  Bus Selector7/7 -> [Traffic25_Yaw]  "<r_zyx z>"
  [Traffic27_YawRate] -> Mux6/7
  Mux1/1 -> To Workspace4/1, [obs_y]
  Bus Selector10/5 -> [Traffic28_Ax]  "<a_0 x>"
  Mux5/1 -> To Workspace5/1, [obs_Vy]
  [Traffic25_Vy] -> Mux5/5
  Constant17/1 -> [route3_waypoint_x]
  Read CM Dict6/1 -> [Traffic21_YawRate]
  [Traffic28_Ax] -> Mux8/8
  Traffic Object10/2 -> Bus Selector10/1
  [Traffic24_Vx] -> Mux2/4
  Bus Selector10/7 -> [Traffic28_Yaw]  "<r_zyx z>"
  [Traffic24_Yaw] -> Mux7/4
  [Traffic23_Yaw] -> Mux7/3
  [Traffic21_Ay] -> Mux9/1
  Read CM Dict16/1 -> [Traffic26_YawRate]
  Bus Selector8/5 -> [Traffic26_Ax]  "<a_0 x>"
  Read CM Dict11/1 -> [Ego_Gloabl_Y]
  Bus Selector9/5 -> [Traffic27_Ax]  "<a_0 x>"
  [Traffic28_Global_Y] -> Mux1/8
  [Traffic22_Yaw] -> Mux7/2
  Mux2/1 -> To Workspace1/1, [obs_Vx]
  Traffic Object6/1 -> Terminator6/1
  [Traffic28_Global_X] -> Mux/8
  Traffic Object4/2 -> Bus Selector4/1
  [Traffic23_YawRate] -> Mux6/3
  [Traffic27_Vy] -> Mux5/7
  Constant19/1 -> [route4_waypoint_x]
  [Traffic21_Global_X] -> Mux/1
  Traffic Object8/1 -> Terminator8/1
  [Traffic25_YawRate] -> Mux6/5
  [Traffic23_Global_X] -> Mux/3
  Constant22/1 -> Traffic Object5/1
  Bus Selector4/1 -> [Traffic22_Global_X]  "<t_0 x>"
  Mux8/1 -> To Workspace3/1, [obs_Ax]
  Constant16/1 -> [route3_waypoint_y]
  [Traffic22_Ay] -> Mux9/2
  Constant21/1 -> [route5_waypoint_x]
  Read CM Dict7/1 -> [Traffic22_YawRate]
  Constant18/1 -> [route4_waypoint_y]
  Bus Selector5/4 -> [Traffic23_Vy]  "<v_0 y>"
  [Traffic25_Vx] -> Mux2/5
  Bus Selector7/3 -> [Traffic25_Vx]  "<v_0 x>"
  Bus Selector3/6 -> [Traffic21_Ay]  "<a_0 y>"
  Constant27/1 -> Traffic Object7/1
  [Traffic26_Yaw] -> Mux7/6
  Constant20/1 -> [route5_waypoint_y]
  Constant8/1 -> Mux4/1
  Bus Selector8/2 -> [Traffic26_Global_Y]  "<t_0 y>"
  Constant9/1 -> Traffic Object4/1
  Subsystem1/1(Traffic_Info) -> [Traffic_Info]
  Read CM Dict15/1 -> [Traffic25_YawRate]
  [Traffic23_Vy] -> Mux5/3
  Bus Selector10/3 -> [Traffic28_Vx]  "<v_0 x>"
  Constant7/1 -> Traffic Object3/1
  [Traffic21_Vx] -> Mux2/1
  Bus Selector7/5 -> [Traffic25_Ax]  "<a_0 x>"
  [Traffic25_Yaw] -> Mux7/5
  Bus Selector4/7 -> [Traffic22_Yaw]  "<r_zyx z>"
  Bus Selector6/3 -> [Traffic24_Vx]  "<v_0 x>"
  [Traffic23_Ax] -> Mux8/3
  Constant13/1 -> [route2_waypoint_y]
  Read CM Dict14/1 -> [Traffic24_YawRate]
  Bus Selector8/6 -> [Traffic26_Ay]  "<a_0 y>"
  Bus Selector3/7 -> [Traffic21_Yaw]  "<r_zyx z>"
  Reshape2/1 -> [Traffic_size]
  Bus Selector8/1 -> [Traffic26_Global_X]  "<t_0 x>"
  Traffic Object5/2 -> Bus Selector5/1
  Bus Selector3/2 -> [Traffic21_Global_Y]  "<t_0 y>"
  [Traffic26_Vy] -> Mux5/6
  Bus Selector6/1 -> [Traffic24_Global_X]  "<t_0 x>"
  [Traffic22_Global_Y] -> Mux1/2
  [Traffic26_YawRate] -> Mux6/6
  [Traffic22_Vy] -> Mux5/2
  [Traffic23_Vx] -> Mux2/3
  [Traffic24_Ay] -> Mux9/4
  Bus Selector3/3 -> [Traffic21_Vx]  "<v_0 x>"
  Bus Selector9/4 -> [Traffic27_Vy]  "<v_0 y>"
  Constant12/1 -> [route1_waypoint_y]
  Bus Selector7/4 -> [Traffic25_Vy]  "<v_0 y>"
  Mux4/1 -> Reshape2/1
  Read CM Dict1/1 -> [Ego_Ax]
  [Ego_Vx] -> Add/2
  [Target_Speed] -> Add/1
